simulink model "open_loop"  (R2012b)
settings: Solver=ode3  StartTime=0.0  StopTime=125  FixedStep=0.001  RelTol=1e-3
values from neighbouring files (symbols this model uses):
  a = D/(8*(t1^2)*(n^2))    [Craneparameters.m]    (also in Craneparameters2.m = 0.428041999052; Craneparameters3.m = 0.428041999052; Craneparameters4.m = 0.5; Craneparameters5.m = 0.428041999052)
  g = 9.81    [Craneparameters.m]    (also in Craneparameters2.m; Craneparameters3.m; Craneparameters4.m; Craneparameters5.m)
  l = 40    [Craneparameters.m]    (also in Craneparameters2.m; Craneparameters3.m; Craneparameters4.m; Craneparameters5.m)
  m = 67.3*10^3    (= 67300)    [Craneparameters.m]    (also in Craneparameters2.m; Craneparameters3.m; Craneparameters4.m; Craneparameters5.m)
  M = 26*10^3    (= 26000)    [Craneparameters.m]    (also in Craneparameters2.m; Craneparameters3.m; Craneparameters4.m; Craneparameters5.m)
  T = 2*pi/w    [Craneparameters.m]    (also in Craneparameters2.m; Craneparameters3.m; Craneparameters4.m; Craneparameters5.m)
  T1 = n*T    [Craneparameters.m]    (also in Craneparameters2.m; Craneparameters3.m; Craneparameters4.m = t1; Craneparameters5.m)
  t1 = T/4    [Craneparameters.m]    (also in Craneparameters2.m; Craneparameters3.m; Craneparameters4.m = round(100*Vmax/a)/100; Craneparameters5.m)
  T2 = n*T+t2    [Craneparameters.m]    (also in Craneparameters2.m; Craneparameters3.m = (n+1)*T; Craneparameters4.m = t1+t2; Craneparameters5.m = (n+1)*T)
  t_total = 2*n*T + t2    [Craneparameters.m]    (also in Craneparameters2.m = t_total2; Craneparameters3.m = 2*(n+1)*T + t2; Craneparameters4.m = T2+t1; Craneparameters5.m = 2*(n+1)*T + t2)
settings Model: Creator=mchusr  LastModifiedBy=mchusr

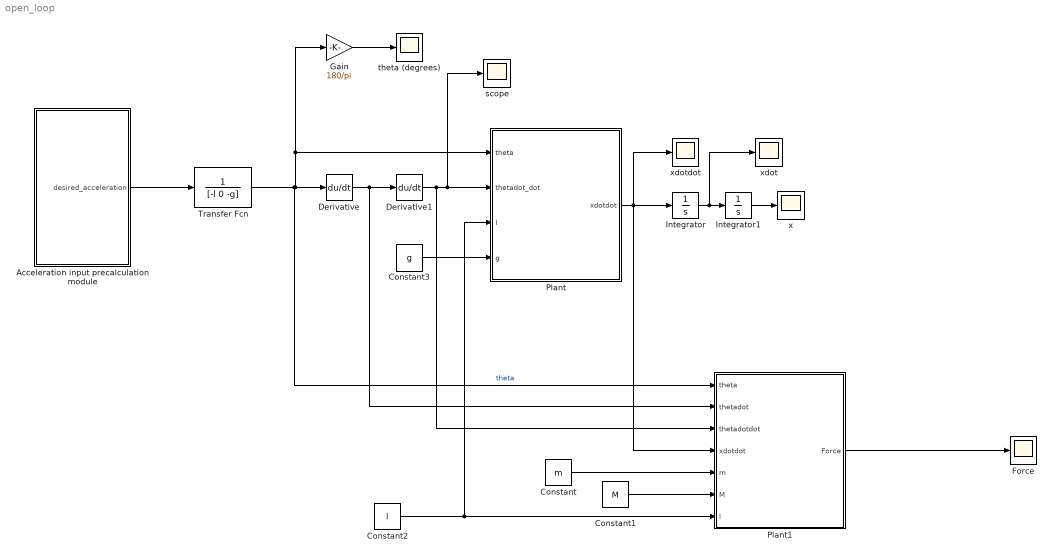
== system open_loop ==
  Acceleration input precalculation module : Subsystem
  Constant : Constant  Value=m
  Constant1 : Constant  Value=M
  Constant2 : Constant  Value=l
  Constant3 : Constant  Value=g
  Derivative : Derivative
  Derivative1 : Derivative
  Force : Scope
      settings: SaveName=Force
  Gain : Gain  Gain=180/pi
  Integrator : Integrator
  Integrator1 : Integrator
  Plant : Subsystem
  Plant1 : Subsystem
  Transfer Fcn : TransferFcn  Denominator=[-l 0 -g]
  scope : Scope
      settings: SaveName=degrees1
  theta (degrees) : Scope
      settings: SaveName=degrees
  x : Scope
      settings: SaveName=position
  xdot : Scope
      settings: SaveName=velocity
  xdotdot : Scope
      settings: TimeRange=105  SaveName=xdotdot
  wires:
  Transfer Fcn/1 -> Gain/1, Plant/1(theta), Derivative/1, Plant1/1(theta)  "theta"
  Derivative/1 -> Plant1/2(thetadot), Derivative1/1
  Derivative1/1 -> Plant1/3(thetadotdot), scope/1, Plant/2(thetadot_dot)
  Plant/1(xdotdot) -> Integrator/1, Plant1/4("xdotdot "), xdotdot/1
  Plant1/1(Force) -> Force/1
  Constant1/1 -> Plant1/6(M)
  Constant/1 -> Plant1/5(m)
  Constant2/1 -> Plant1/7(l), Plant/3(l)
  Constant3/1 -> Plant/4(g)
  Integrator/1 -> xdot/1, Integrator1/1
  Integrator1/1 -> x/1
  Gain/1 -> theta (degrees)/1
  Acceleration input precalculation module/1(desired_acceleration) -> Transfer Fcn/1

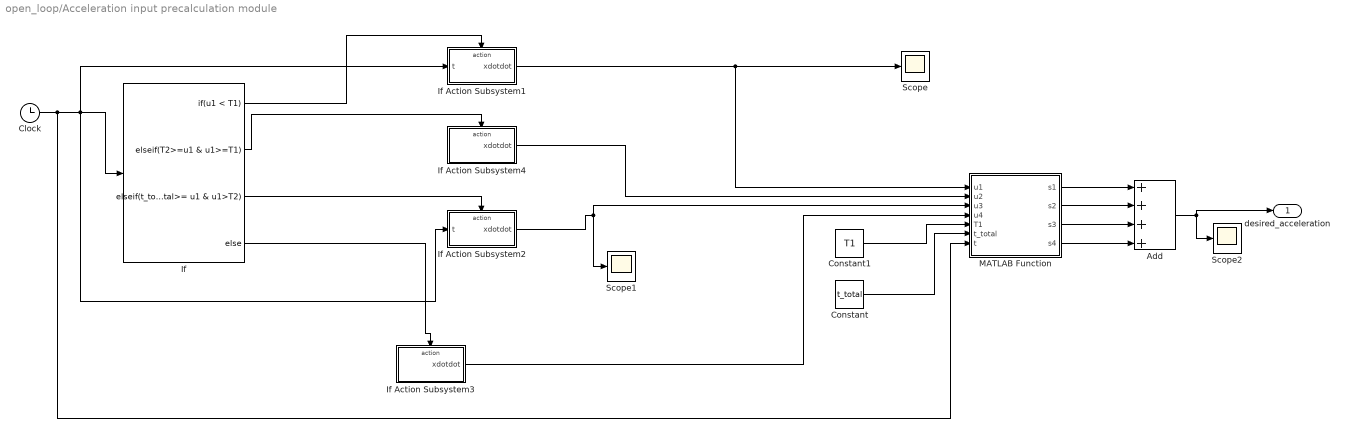
== system open_loop/Acceleration input precalculation module ==
  Add : Sum  Inputs=++++
  Clock : Clock
  Constant : Constant  Value=t_total
  Constant1 : Constant  Value=T1
  If : If  IfExpression=u1 < T1  ElseIfExpressions=T2>=u1 & u1>=T1, t_total>= u1 & u1>T2  ZeroCross=off
  If Action Subsystem1 : Subsystem  TreatAsAtomicUnit=on
  If Action Subsystem2 : Subsystem  TreatAsAtomicUnit=on
  If Action Subsystem3 : Subsystem  TreatAsAtomicUnit=on
  If Action Subsystem4 : Subsystem  TreatAsAtomicUnit=on
  MATLAB Function : MATLAB Function  TreatAsAtomicUnit=on
  Scope : Scope
      settings: SaveName=ScopeData4
  Scope1 : Scope
      settings: SaveName=ScopeData5
  Scope2 : Scope
      settings: SaveName=ScopeData6
  desired_acceleration : Outport
  wires:
  If/1 -> If Action Subsystem1/Action
  If/2 -> If Action Subsystem4/Action
  If/3 -> If Action Subsystem2/Action
  Clock/1 -> MATLAB Function/7(t), If Action Subsystem1/1(t), If Action Subsystem2/1(t), If/1
  Add/1 -> Scope2/1, desired_acceleration/1
  If Action Subsystem4/1(xdotdot) -> MATLAB Function/2(u2)
  If Action Subsystem2/1(xdotdot) -> MATLAB Function/3(u3), Scope1/1
  If Action Subsystem3/1(xdotdot) -> MATLAB Function/4(u4)
  If/4 -> If Action Subsystem3/Action
  If Action Subsystem1/1(xdotdot) -> MATLAB Function/1(u1), Scope/1
  MATLAB Function/1(s1) -> Add/1
  MATLAB Function/2(s2) -> Add/2
  MATLAB Function/3(s3) -> Add/3
  MATLAB Function/4(s4) -> Add/4
  Constant1/1 -> MATLAB Function/5(T1)
  Constant/1 -> MATLAB Function/6(t_total)

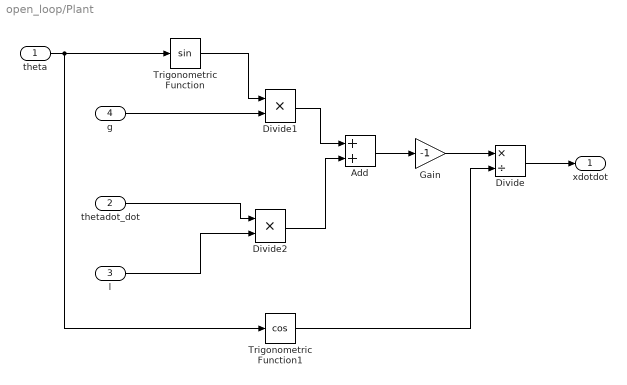
== system open_loop/Plant ==
  theta : Inport
  thetadot_dot : Inport  Port=2
  l : Inport  Port=3
  g : Inport  Port=4
  Add : Sum
  Divide : Product  Inputs=*/
  Divide1 : Product  Inputs=**
  Divide2 : Product  Inputs=**
  Gain : Gain  Gain=-1
  Trigonometric Function : Trigonometry
  Trigonometric Function1 : Trigonometry  Operator=cos
  xdotdot : Outport
  wires:
  theta/1 -> Trigonometric Function/1, Trigonometric Function1/1
  Trigonometric Function/1 -> Divide1/1
  g/1 -> Divide1/2
  Divide1/1 -> Add/1
  thetadot_dot/1 -> Divide2/1
  l/1 -> Divide2/2
  Divide2/1 -> Add/2
  Add/1 -> Gain/1
  Gain/1 -> Divide/1
  Trigonometric Function1/1 -> Divide/2
  Divide/1 -> xdotdot/1

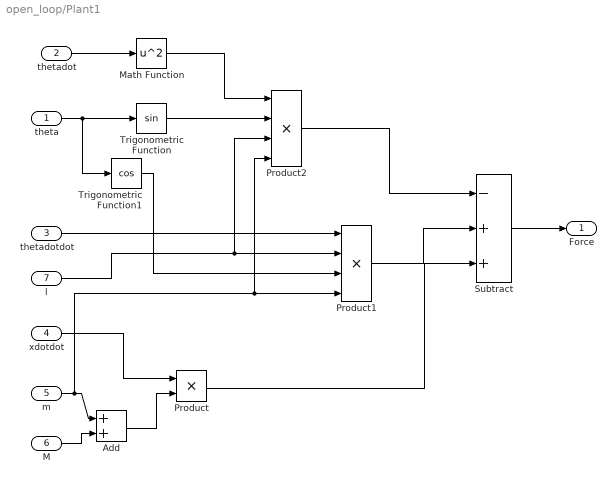
== system open_loop/Plant1 ==
  theta : Inport
  thetadot : Inport  Port=2
  thetadotdot : Inport  Port=3
  "xdotdot " : Inport  Port=4
  m : Inport  Port=5
  M : Inport  Port=6
  l : Inport  Port=7
  Add : Sum
  Math Function : Math  Operator=square  SaturateOnIntegerOverflow=on
  Product : Product  RndMeth=Zero
  Product1 : Product  Inputs=4  RndMeth=Zero
  Product2 : Product  Inputs=4  RndMeth=Zero
  Subtract : Sum  Inputs=-++
  Trigonometric Function : Trigonometry
  Trigonometric Function1 : Trigonometry  Operator=cos
  Force : Outport
  wires:
  Subtract/1 -> Force/1
  theta/1 -> Trigonometric Function1/1, Trigonometric Function/1
  m/1 -> Product2/4, Product1/4, Add/1
  M/1 -> Add/2
  "xdotdot "/1 -> Product/1
  Add/1 -> Product/2
  thetadotdot/1 -> Product1/1
  l/1 -> Product2/3, Product1/2
  Trigonometric Function1/1 -> Product1/3
  thetadot/1 -> Math Function/1
  Math Function/1 -> Product2/1
  Trigonometric Function/1 -> Product2/2
  Product2/1 -> Subtract/1
  Product1/1 -> Subtract/2
  Product/1 -> Subtract/3

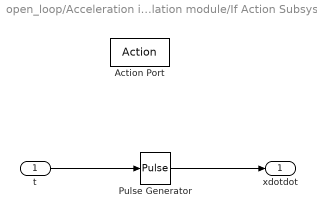
== system open_loop/Acceleration input precalculation module/If Action Subsystem1 ==
  t : Inport
  Action Port : ActionPort  ActionType=then
  Pulse Generator : DiscretePulseGenerator  PulseType=Time based  TimeSource=Use external signal  Amplitude=a  Period=T/2  PulseWidth=50  SampleTime=0.001
  xdotdot : Outport
  wires:
  Pulse Generator/1 -> xdotdot/1
  t/1 -> Pulse Generator/1

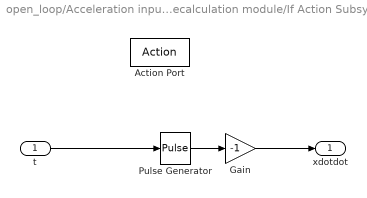
== system open_loop/Acceleration input precalculation module/If Action Subsystem2 ==
  t : Inport
  Action Port : ActionPort  ActionType=elseif
  Gain : Gain  Gain=-1
  Pulse Generator : DiscretePulseGenerator  PulseType=Time based  TimeSource=Use external signal  Amplitude=a  Period=T/2  PulseWidth=50  PhaseDelay=T2+t1  SampleTime=0.001
  xdotdot : Outport
  wires:
  t/1 -> Pulse Generator/1
  Pulse Generator/1 -> Gain/1
  Gain/1 -> xdotdot/1

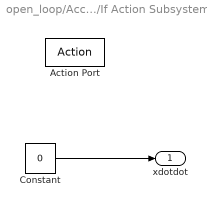
== system open_loop/Acceleration input precalculation module/If Action Subsystem3 ==
  Action Port : ActionPort  ActionType=else
  Constant : Constant  Value=0
  xdotdot : Outport
  wires:
  Constant/1 -> xdotdot/1

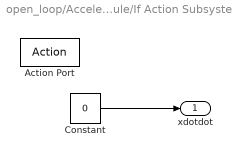
== system open_loop/Acceleration input precalculation module/If Action Subsystem4 ==
  Action Port : ActionPort  ActionType=elseif
  Constant : Constant  Value=0
  xdotdot : Outport
  wires:
  Constant/1 -> xdotdot/1

== matlab function open_loop/Acceleration input precalculation module/MATLAB Function ==
  data: u1 input; s1 output; u2 input; u3 input; u4 input; T1 input; t_total input; s2 output; s3 output; s4 output; t input
function [s1, s2, s3, s4] = filter(u1, u2, u3, u4, T1, t_total, t)

if t<T1
    s1 = u1;
else
    s1=0;
end



if t<t_total
    s3 = u3;
else
    s3=0;
end

s2=u2;

s4=u4;




end
